simulink model "Prob_7_model"  (R2016a)
settings: Solver=FixedStepDiscrete  StartTime=0.0  StopTime=10.0  RelTol=1e-3
libraries: simulink x1
settings Model: Creator=Admin  LastModifiedBy=Admin

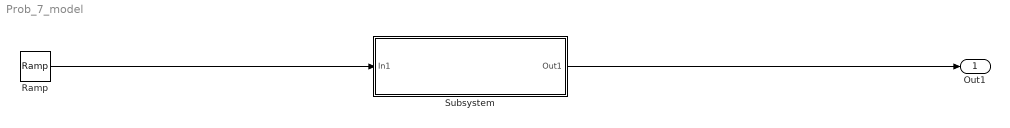
== system Prob_7_model ==
  Ramp : simulink/Sources/Ramp  slope=1  start=0  X0=0
  Subsystem : Subsystem
  Out1 : Outport
  wires:
  Ramp/1 -> Subsystem/1(In1)
  Subsystem/1(Out1) -> Out1/1

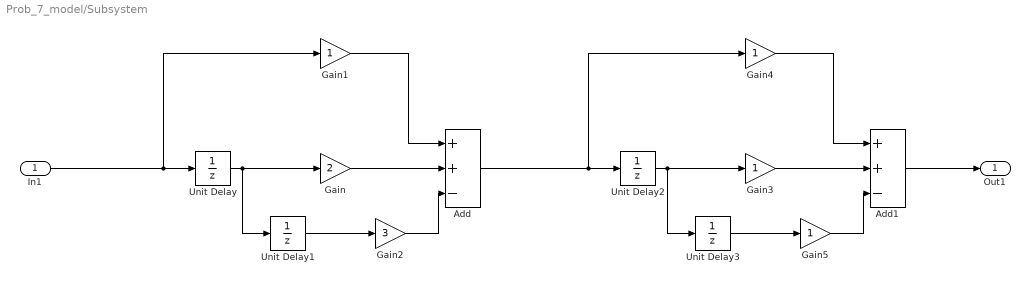
== system Prob_7_model/Subsystem ==
  In1 : Inport
  Add : Sum  Inputs=++-
  Add1 : Sum  Inputs=++-
  Gain : Gain  Gain=2
  Gain{1,3..5} (4 alike) : Gain
  Gain2 : Gain  Gain=3
  Unit Delay{,1..3} (4 alike) : UnitDelay  SampleTime=-1
  Out1 : Outport
  wires:
  Gain1/1 -> Add/1
  In1/1 -> Unit Delay/1, Gain1/1
  Unit Delay/1 -> Unit Delay1/1, Gain/1
  Gain/1 -> Add/2
  Unit Delay2/1 -> Unit Delay3/1, Gain3/1
  Unit Delay1/1 -> Gain2/1
  Gain2/1 -> Add/3
  Add1/1 -> Out1/1
  Unit Delay3/1 -> Gain5/1
  Add/1 -> Unit Delay2/1, Gain4/1
  Gain4/1 -> Add1/1
  Gain3/1 -> Add1/2
  Gain5/1 -> Add1/3
